simulink model "focVelocityEncoder"  (R2020a)
settings: configuration reference "EC" (kept outside this file)
model workspace (MAT data in the model file):
  PolePairs = 4
  activeLoop = 1
  statusAutotuner = 0
undefined symbols (not defined in the file): adcTransducerVoltAtZeroAmpere, adcTransducerVoltPerAmpere, DiscIntNeverNeededParam, encoderCalibrationDuration, encoderCalibrationVoltage, encoderCountPerRevolution, inverterBusVoltage, inverterCurrentMax, paramCurrentControlI, paramCurrentControlP, paramOpenLoopVelocityAcceleration, paramOpenLoopVelocityToVoltsBias, paramOpenLoopVelocityToVoltsScalar, paramOverCurrentEnable, paramVelocityControlI, paramVelocityControlP, pwmComparePerVolt, pwmCounterMax, sampleTimeCurrentControl
libraries: mcbcontrolslib x12, simulink x7, mcbpositiondecoderlib x4, focautotunershared x1
settings Model: DataDictionary=controllerData.sldd  EnableAccessToBaseWorkspace=off  ParameterArgumentNames=PolePairs,activeLoop,statusAutotuner  OrderedModelArguments=off  Creator=The MathWorks, Inc.  LastModifiedBy=manuel.fedou
settings ConfigSetRef: SourceName=EC

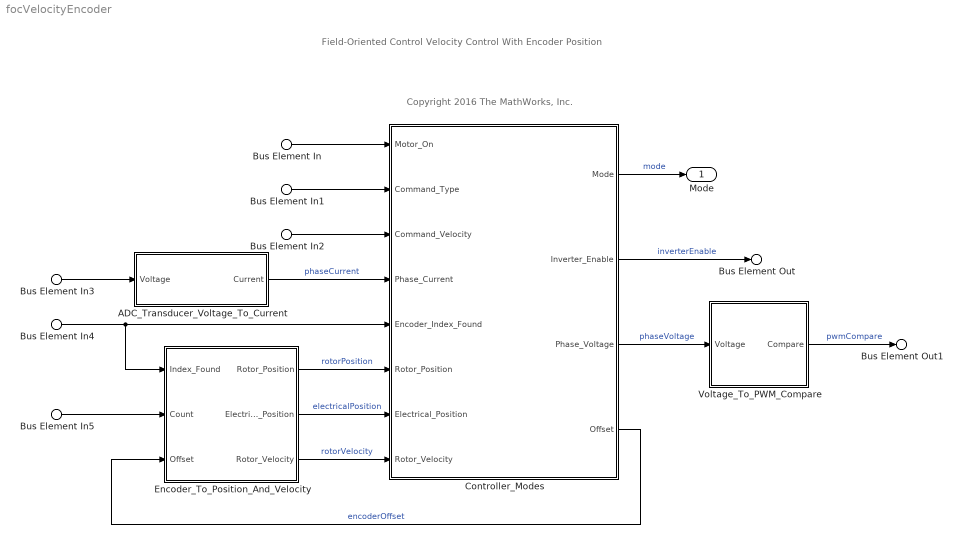
== system focVelocityEncoder ==
  note: Field-Oriented Control
      | Velocity Control With Encoder Position
  note: Copyright 2016 The MathWorks, Inc.
  Bus Element In : Inport  PortName=inputs  Element=motorOn
  Bus Element In1 : Inport  PortName=inputs  Element=commandType
  Bus Element In2 : Inport  PortName=inputs  Element=velocityCommand
  Bus Element In3 : Inport  Port=2  PortName=feedback  Element=transducerVoltage
  Bus Element In4 : Inport  Port=2  PortName=feedback  Element=encoderIndexFound
  Bus Element In5 : Inport  Port=2  PortName=feedback  Element=encoderCount
  ADC_Transducer_Voltage_To_Current : Subsystem
  Controller_Modes : Subsystem
  Encoder_To_Position_And_Velocity : Subsystem  VariantControl=isMCB == 1
  Voltage_To_PWM_Compare : Subsystem
  Mode : Outport  PortDimensions=1  VectorParamsAs1DForOutWhenUnconnected=off
  Bus Element Out : Outport  Port=2  PortName=commands  Element=inverterEnable
  Bus Element Out1 : Outport  Port=2  PortName=commands  Element=pwmCompare
  wires:
  ADC_Transducer_Voltage_To_Current/1(Current) -> Controller_Modes/4(Phase_Current)  "phaseCurrent"
  Controller_Modes/4(Offset) -> Encoder_To_Position_And_Velocity/3(Offset)  "encoderOffset"
  Bus Element In4/1 -> Encoder_To_Position_And_Velocity/1(Index_Found), Controller_Modes/5(Encoder_Index_Found)
  Voltage_To_PWM_Compare/1(Compare) -> Bus Element Out1/1  "pwmCompare"
  Bus Element In3/1 -> ADC_Transducer_Voltage_To_Current/1(Voltage)
  Controller_Modes/1(Mode) -> Mode/1  "mode"
  Controller_Modes/3(Phase_Voltage) -> Voltage_To_PWM_Compare/1(Voltage)  "phaseVoltage"
  Controller_Modes/2(Inverter_Enable) -> Bus Element Out/1  "inverterEnable"
  Bus Element In5/1 -> Encoder_To_Position_And_Velocity/2(Count)
  Encoder_To_Position_And_Velocity/1(Rotor_Position) -> Controller_Modes/6(Rotor_Position)  "rotorPosition"
  Encoder_To_Position_And_Velocity/2(Electrical_Position) -> Controller_Modes/7(Electrical_Position)  "electricalPosition"
  Encoder_To_Position_And_Velocity/3(Rotor_Velocity) -> Controller_Modes/8(Rotor_Velocity)  "rotorVelocity"
  Bus Element In1/1 -> Controller_Modes/2(Command_Type)
  Bus Element In/1 -> Controller_Modes/1(Motor_On)
  Bus Element In2/1 -> Controller_Modes/3(Command_Velocity)

== system focVelocityEncoder/ADC_Transducer_Voltage_To_Current ==
  note: ADC Transducer Voltage to Current
  Voltage : Inport
  Add : Sum  Inputs=+-
  Bias_To_Remove : Constant  Value=adcTransducerVoltAtZeroAmpere  OutDataTypeStr=Inherit: Inherit via back propagation  SampleTime=-1
  Divide : Product  Inputs=*/
  Scalar : Constant  Value=adcTransducerVoltPerAmpere  OutDataTypeStr=Inherit: Inherit via back propagation  SampleTime=-1
  Current : Outport  VectorParamsAs1DForOutWhenUnconnected=off
  wires:
  Voltage/1 -> Add/1
  Add/1 -> Divide/1
  Scalar/1 -> Divide/2
  Divide/1 -> Current/1
  Bias_To_Remove/1 -> Add/2

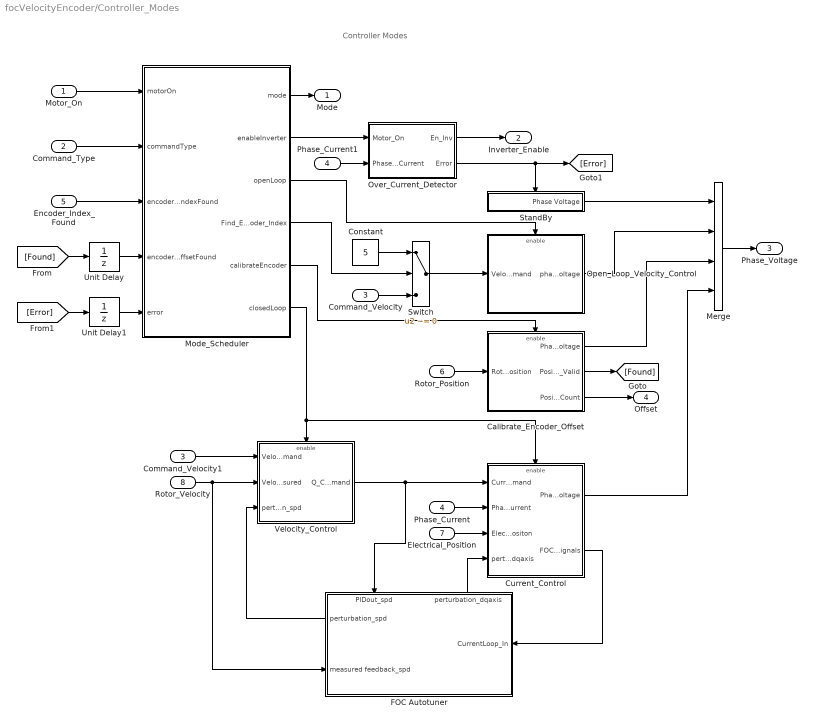
== system focVelocityEncoder/Controller_Modes ==
  note: Controller Modes
  Motor_On : Inport
  Command_Type : Inport  Port=2
  Command_Velocity : Inport  Port=3
  Phase_Current : Inport  Port=4
  Encoder_Index_Found : Inport  Port=5
  Rotor_Position : Inport  Port=6
  Electrical_Position : Inport  Port=7
  Rotor_Velocity : Inport  Port=8
  Calibrate_Encoder_Offset : Subsystem
      mask Display: fprintf('Calibrate\nEncoder\nOffset')
  Command_Velocity1 : InportShadow  Port=3
  Constant : Constant  Value=5  OutDataTypeStr=Inherit: Inherit via back propagation  SampleTime=-1
  Current_Control : Subsystem
      mask Display: fprintf('Current\nControl')
  FOC Autotuner : Subsystem  Variant=on  VariantControlMode=Label  VariantControl=Choice  LabelModeActiveChoice=dummyVariant
      settings: PortSchema="{\"entries\":[{\"content\":{\"sides\":[{\"content\":{\"connectorIds\":[\"Out2\",\"In1\"]},\"type\":\"ConnectorPlacement.EquallySpacedRectSide\",\"uuid\":\"a8b69d11-b8b6-4c45-a37c-f2894d64c9bb\"},{\"content\":{\"connectorIds\":[\"In3\"],\"side\":\"RIGHT\"},\"type\":\"ConnectorPlacement.EquallySpacedRectSide\",\"uuid\":\"22efc6fa-b445-4d82-b4a6-fe483b816bd6\"},{\"content\":{\"connectorIds\":[\"In2\",\"Out1\"],\"side\":\"TOP\"},\"type\":\"ConnectorPlacement.EquallySpacedRectSide\",\"uuid\":\"13837f3f-03ad-4a4a-a1cf-81e26a9a881f\"}]},\"type\":\"ConnectorPlacement.EquallySpacedConnector\",\"uuid\":\"91c3fe0f-f3e7-4ad7-9fa7-cccbc8809dba\"}],\"packageUris\":[\"http://schema.mathworks.com/mf0/Connector/19700101\"],\"version\":\"1.0\"}"
  Merge : Merge  Inputs=4
      mask Display: fprintf(' ')
  Mode_Scheduler : Stateflow chart  TreatAsAtomicUnit=on
  Open_Loop_Velocity_Control : Subsystem  TreatAsAtomicUnit=on
      settings: RTWFcnNameOpts=User specified  FunctionInterfaceSpec=Allow arguments (Optimized)
      mask Display: fprintf('Open Loop\nVelocity\nControl')
  Over_Current_Detector : Subsystem  TreatAsAtomicUnit=on
      mask Display: fprintf('Detect\nOvercurrent')
  Phase_Current1 : InportShadow  Port=4
  StandBy : Subsystem  Description=Stand By mode for controller outputs constant phase voltages.  TreatAsAtomicUnit=on
      mask Display: fprintf('Disabled')
  Switch : Switch  Criteria=u2 ~= 0
  Unit Delay : UnitDelay  SampleTime=-1  HasFrameUpgradeWarning=on
  Unit Delay1 : UnitDelay  SampleTime=-1  HasFrameUpgradeWarning=on
  Velocity_Control : Subsystem
      mask Display: fprintf('Velocity\nControl')
  Mode : Outport  VectorParamsAs1DForOutWhenUnconnected=off
  Inverter_Enable : Outport  Port=2  VectorParamsAs1DForOutWhenUnconnected=off
  Phase_Voltage : Outport  Port=3  VectorParamsAs1DForOutWhenUnconnected=off
  Offset : Outport  Port=4  VectorParamsAs1DForOutWhenUnconnected=off
  wires:
  Calibrate_Encoder_Offset/2(Position_At_Zero_Count_Valid) -> [Found]
  Phase_Current1/1 -> Over_Current_Detector/2(Phase_Current)
  Mode_Scheduler/2(" enableInverter") -> Over_Current_Detector/1(Motor_On)
  Merge/1 -> Phase_Voltage/1
  Calibrate_Encoder_Offset/3(Position_At_Zero_Count) -> Offset/1
  Rotor_Position/1 -> Calibrate_Encoder_Offset/1(Rotor_Position)
  Calibrate_Encoder_Offset/1(Phase_Voltage) -> Merge/3
  StandBy/1(Phase Voltage) -> Merge/1
  Mode_Scheduler/5(" calibrateEncoder") -> Calibrate_Encoder_Offset/Enable
  Switch/1 -> Open_Loop_Velocity_Control/1(Velocity_Command)
  Open_Loop_Velocity_Control/1(phase_voltage) -> Merge/2
  Current_Control/1(Phase_Voltage) -> Merge/4
  Phase_Current/1 -> Current_Control/2(Phase_Current)
  Electrical_Position/1 -> Current_Control/3(Electrical_Positon)
  Mode_Scheduler/3(" openLoop") -> Open_Loop_Velocity_Control/Enable
  Rotor_Velocity/1 -> Velocity_Control/2(Velocity_Measured), FOC Autotuner/1(measured feedback_spd)
  Over_Current_Detector/1(En_Inv) -> Inverter_Enable/1
  Command_Type/1 -> Mode_Scheduler/2(commandType)
  Motor_On/1 -> Mode_Scheduler/1(motorOn)
  [Error] -> Unit Delay1/1
  [Found] -> Unit Delay/1
  Encoder_Index_Found/1 -> Mode_Scheduler/3(encoderIndexFound)
  Mode_Scheduler/1(mode) -> Mode/1
  FOC Autotuner/1(perturbation_dqaxis) -> Current_Control/4(perturbation_dqaxis)
  Current_Control/2(FOC_Autotuner_Signals) -> FOC Autotuner/3(CurrentLoop_In)
  FOC Autotuner/2(perturbation_spd) -> Velocity_Control/3(perturbation_spd)
  Velocity_Control/1(Q_Current_Command) -> Current_Control/1(Current_Command), FOC Autotuner/2(PIDout_spd)
  Mode_Scheduler/4(" Find_Encoder_Index") -> Switch/2
  Command_Velocity/1 -> Switch/3
  Constant/1 -> Switch/1
  Over_Current_Detector/2(Error) -> StandBy/Enable, [Error]
  Command_Velocity1/1 -> Velocity_Control/1(Velocity_Command)
  Unit Delay/1 -> Mode_Scheduler/4(encoderOffsetFound)
  Unit Delay1/1 -> Mode_Scheduler/5(error)
  Mode_Scheduler/6(" closedLoop") -> Velocity_Control/Enable, Current_Control/Enable

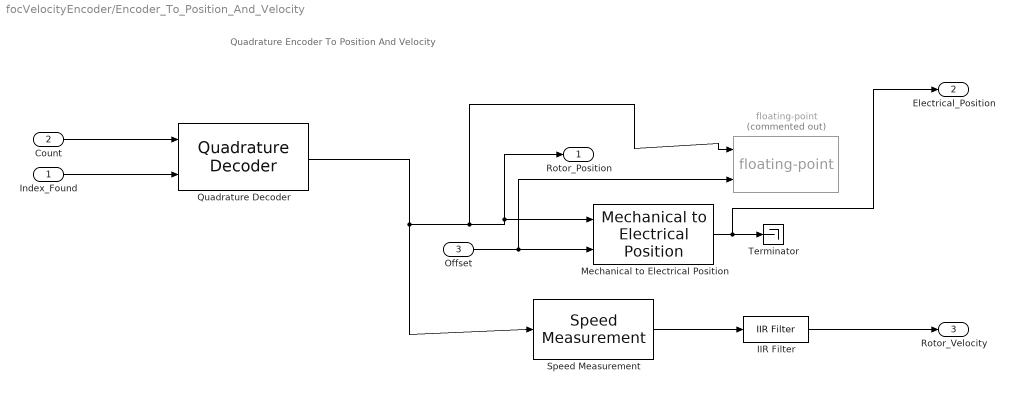
== system focVelocityEncoder/Encoder_To_Position_And_Velocity ==
  note: Quadrature Encoder To Position And Velocity
  Index_Found : Inport
  Count : Inport  Port=2
  Offset : Inport  Port=3
  IIR Filter : mcbcontrolslib/IIR Filter  Filter_constant=0.01
      settings: SourceProductBaseCode=MT
  Mechanical to Electrical Position : mcbpositiondecoderlib/Mechanical to Electrical Position  LabelModeActiveChoice=floating-point  NrPP=7  selectedRange=Radians  MechOfstInputType=Input port  mechOffsetIn=0  maxAngleIn=2*pi  InputDataType=single  VariantSelect=floating-point
      settings: SourceProductBaseCode=MT
  Quadrature Decoder : mcbpositiondecoderlib/Quadrature Decoder  EncoderSlitsPerRevolution=1024  EncoderCountsPerSlit=4  CounterSize=16 bits  ExternalIndexCount=on  PositionUnit=Radians  PositionDataType=single
      settings: SourceProductBaseCode=MT
  Speed Measurement : mcbpositiondecoderlib/Speed Measurement  PositionUnit=Radians  SpeedCalculationMode=Maximum application speed  SampleTimeAsync=0.0002  MaximumApplicationSpeed=5000  SpeedResolution=3  DelayLength=29  MaximumMeasurableSpeed=5000  MeasurableSpeedResolution=2.3283e-06  SpeedUnit=Radians/Sec  PerUnitSpeed=1000  SpeedDataType=single
      settings: SourceProductBaseCode=MT
  Terminator : Terminator
  floating-point : mcbpositiondecoderlib/Mechanical to Electrical Position/floating-point  Commented=on  SystemSampleTime=-1  VariantControl=floating-point  Latency=0  AutoFrameSizeCalculation=off
      settings: SourceProductBaseCode=MT
  Rotor_Position : Outport  VectorParamsAs1DForOutWhenUnconnected=off
  Electrical_Position : Outport  Port=2  VectorParamsAs1DForOutWhenUnconnected=off
  Rotor_Velocity : Outport  Port=3  VectorParamsAs1DForOutWhenUnconnected=off
  wires:
  Index_Found/1 -> Quadrature Decoder/2
  Count/1 -> Quadrature Decoder/1
  Speed Measurement/1 -> IIR Filter/1
  IIR Filter/1 -> Rotor_Velocity/1
  Offset/1 -> floating-point/2, Mechanical to Electrical Position/2
  Quadrature Decoder/1 -> Mechanical to Electrical Position/1, Rotor_Position/1, floating-point/1, Speed Measurement/1
  Mechanical to Electrical Position/1 -> Electrical_Position/1, Terminator/1

== system focVelocityEncoder/Voltage_To_PWM_Compare ==
  note: Voltage To PWM Compare
  Voltage : Inport
  Bias1 : Bias  Bias=pwmCounterMax/2
  Data_Type_Conversion : DataTypeConversion  OutDataTypeStr=uint16  LockScale=on
  Saturation : Saturate  UpperLimit=pwmCounterMax  LowerLimit=0
      settings: AttributesFormatString=|
      | --------------------------------
      | Upper Limit = %<UpperLimit>
      | Lower Limit = %<LowerLimit>
  Slope : Gain  Gain=pwmComparePerVolt
      settings: AttributesFormatString=|
      | ----------------------------------------
      | Gain = %<Gain>
  Compare : Outport  VectorParamsAs1DForOutWhenUnconnected=off
  wires:
  Saturation/1 -> Data_Type_Conversion/1
  Voltage/1 -> Slope/1  "phaseVoltage"
  Data_Type_Conversion/1 -> Compare/1  "pwmCompare"
  Slope/1 -> Bias1/1
  Bias1/1 -> Saturation/1

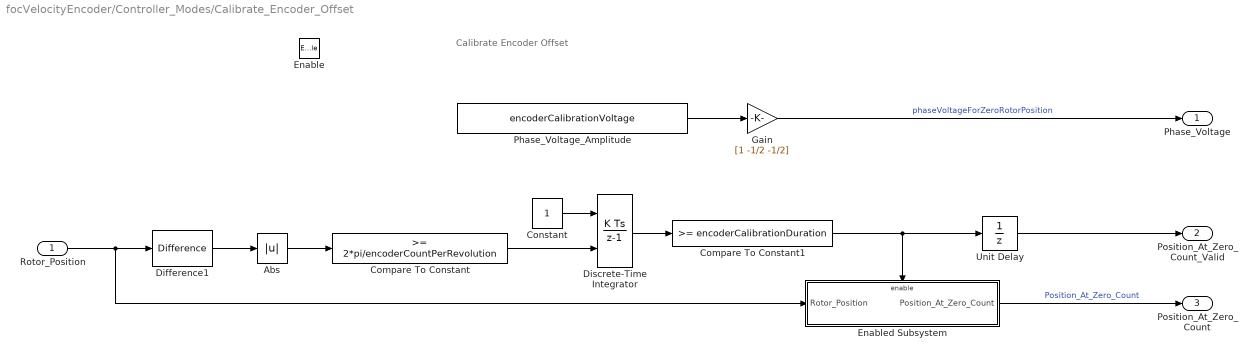
== system focVelocityEncoder/Controller_Modes/Calibrate_Encoder_Offset ==
  note: Calibrate Encoder Offset
  Rotor_Position : Inport  PortDimensions=1  Interpolate=off
  Enable : EnablePort  StatesWhenEnabling=reset
      settings: AttributesFormatString=|
      | ----------------------------------------
      | States when enabling = %<StatesWhenEnabling>
  Abs : Abs
  Compare To Constant : simulink/Logic and Bit Operations/Compare To Constant  relop=>=  const=2*pi/encoderCountPerRevolution  OutDataTypeStr=boolean
  Compare To Constant1 : simulink/Logic and Bit Operations/Compare To Constant  relop=>=  const=encoderCalibrationDuration  OutDataTypeStr=boolean
  Constant : Constant
  Difference1 : simulink/Discrete/Difference  ICPrevInput=0.0  OutMin=[]  OutMax=[]  OutDataType=fixdt(1, 16)  OutScaling=2^-10  DoSatur=off
  Discrete-Time Integrator : DiscreteIntegrator  ExternalReset=rising  SampleTime=-1  ICPrevOutput=DiscIntNeverNeededParam  ICPrevScaledInput=DiscIntNeverNeededParam
  Enabled Subsystem : Subsystem  TreatAsAtomicUnit=on
  Gain : Gain  Gain=[1 -1/2 -1/2]
      settings: AttributesFormatString=|
      | ----------------------------------
      | Gain = %<Gain>
  Phase_Voltage_Amplitude : Constant  Value=encoderCalibrationVoltage  OutDataTypeStr=Inherit: Inherit via back propagation
  Unit Delay : UnitDelay  SampleTime=-1  HasFrameUpgradeWarning=on
  Phase_Voltage : Outport  PortDimensions=3  SourceOfInitialOutputValue=Input signal  InitialOutput=0  VectorParamsAs1DForOutWhenUnconnected=off
  Position_At_Zero_Count_Valid : Outport  Port=2  OutputWhenDisabled=reset  InitialOutput=0  VectorParamsAs1DForOutWhenUnconnected=off
  Position_At_Zero_Count : Outport  Port=3  SourceOfInitialOutputValue=Input signal  VectorParamsAs1DForOutWhenUnconnected=off
  wires:
  Unit Delay/1 -> Position_At_Zero_Count_Valid/1
  Enabled Subsystem/1(Position_At_Zero_Count) -> Position_At_Zero_Count/1  "Position_At_Zero_Count"
  Discrete-Time Integrator/1 -> Compare To Constant1/1
  Constant/1 -> Discrete-Time Integrator/1
  Abs/1 -> Compare To Constant/1
  Difference1/1 -> Abs/1
  Compare To Constant/1 -> Discrete-Time Integrator/2
  Gain/1 -> Phase_Voltage/1  "phaseVoltageForZeroRotorPosition"
  Phase_Voltage_Amplitude/1 -> Gain/1
  Rotor_Position/1 -> Enabled Subsystem/1(Rotor_Position), Difference1/1
  Compare To Constant1/1 -> Unit Delay/1, Enabled Subsystem/Enable

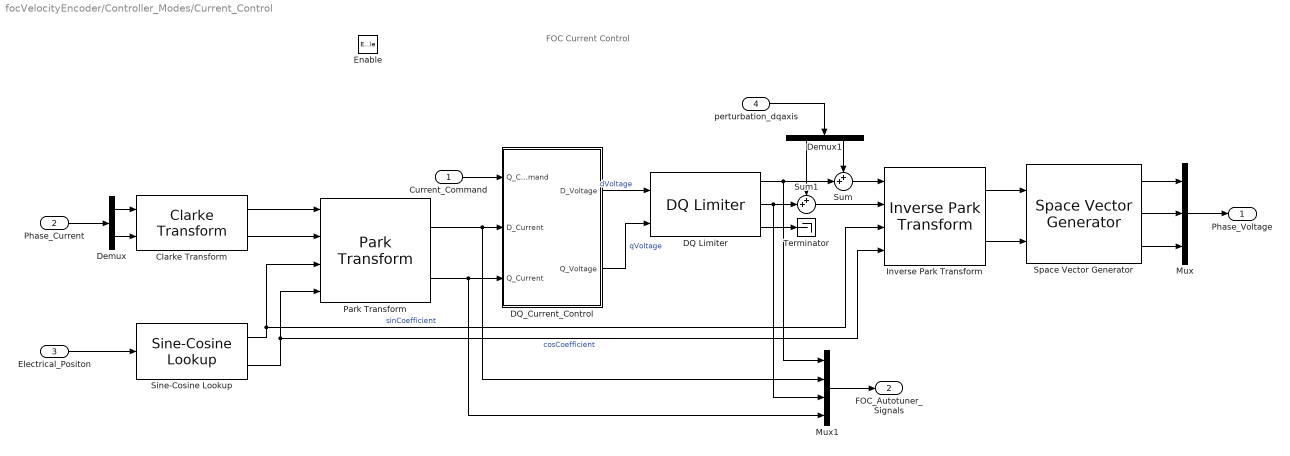
== system focVelocityEncoder/Controller_Modes/Current_Control ==
  note: FOC Current Control
  Current_Command : Inport
  Phase_Current : Inport  Port=2
  Electrical_Positon : Inport  Port=3
  perturbation_dqaxis : Inport  Port=4
  Enable : EnablePort  StatesWhenEnabling=reset
      settings: AttributesFormatString=|
      | ----------------------------------------
      | States when enabling = %<StatesWhenEnabling>
  Clarke Transform : mcbcontrolslib/Clarke Transform  VariantControl=Variant2
  DQ Limiter : mcbcontrolslib/DQ Limiter  Vmax=inverterBusVoltage/sqrt(3)
      settings: SourceProductBaseCode=MT
  DQ_Current_Control : Subsystem
  Demux : Demux  Outputs=2
  Demux1 : Demux  Outputs=2
  Inverse Park Transform : mcbcontrolslib/Inverse Park Transform  AxisAlignment=D-axis
  Mux : Mux  Inputs=3
  Mux1 : Mux
  Park Transform : mcbcontrolslib/Park Transform  AxisAlignment=D-axis
      settings: SourceProductBaseCode=MT
  Sine-Cosine Lookup : mcbcontrolslib/Sine-Cosine Lookup  AngleInput=Radians  N_points=1024
      settings: SourceProductBaseCode=MT
  Space Vector Generator : mcbcontrolslib/Space Vector Generator
      settings: SourceProductBaseCode=MT
  Sum : Sum  Inputs=++|
  Sum1 : Sum  Inputs=++|
  Terminator : Terminator
  Phase_Voltage : Outport  SourceOfInitialOutputValue=Input signal  VectorParamsAs1DForOutWhenUnconnected=off
  FOC_Autotuner_Signals : Outport  Port=2  VectorParamsAs1DForOutWhenUnconnected=off
  wires:
  Park Transform/2 -> Mux1/4, DQ_Current_Control/3(Q_Current)
  Park Transform/1 -> Mux1/2, DQ_Current_Control/2(D_Current)
  Inverse Park Transform/2 -> Space Vector Generator/2
  Inverse Park Transform/1 -> Space Vector Generator/1
  Clarke Transform/2 -> Park Transform/2
  Clarke Transform/1 -> Park Transform/1
  Mux/1 -> Phase_Voltage/1
  Electrical_Positon/1 -> Sine-Cosine Lookup/1
  Sine-Cosine Lookup/2 -> Inverse Park Transform/4, Park Transform/4  "cosCoefficient"
  Sine-Cosine Lookup/1 -> Inverse Park Transform/3, Park Transform/3  "sinCoefficient"
  Demux/1 -> Clarke Transform/1
  Demux/2 -> Clarke Transform/2
  Phase_Current/1 -> Demux/1
  Space Vector Generator/1 -> Mux/1
  Space Vector Generator/2 -> Mux/2
  Space Vector Generator/3 -> Mux/3
  DQ_Current_Control/1(D_Voltage) -> DQ Limiter/1  "dVoltage"
  DQ_Current_Control/2(Q_Voltage) -> DQ Limiter/2  "qVoltage"
  DQ Limiter/3 -> Terminator/1
  Sum/1 -> Inverse Park Transform/1
  DQ Limiter/1 -> Mux1/1, Sum/2
  DQ Limiter/2 -> Mux1/3, Sum1/2
  Sum1/1 -> Inverse Park Transform/2
  Demux1/1 -> Sum1/1
  Demux1/2 -> Sum/1
  perturbation_dqaxis/1 -> Demux1/1
  Mux1/1 -> FOC_Autotuner_Signals/1
  Current_Command/1 -> DQ_Current_Control/1(Q_Command)

== system focVelocityEncoder/Controller_Modes/FOC Autotuner ==
  measured feedback_spd : Inport
  PIDout_spd : Inport  Port=2
  CurrentLoop_In : Inport  Port=3
  Autotuner : Subsystem  VariantControl=autotunerVariant
  Dummy : Subsystem  VariantControl=dummyVariant
  perturbation_dqaxis : Outport
  perturbation_spd : Outport  Port=2

== system focVelocityEncoder/Controller_Modes/Open_Loop_Velocity_Control ==
  note: Open Loop Velocity Control
  Velocity_Command : Inport
  Enable : EnablePort  StatesWhenEnabling=reset
      settings: AttributesFormatString=|
      | ----------------------------------------
      | States when enabling = %<StatesWhenEnabling>
  3-Phase Sine Voltage Generator : mcbcontrolslib/3-Phase Sine Voltage Generator  AngleInput=Radians  N_points=1024
      settings: SourceProductBaseCode=MT
  Mux : Mux  Inputs=3
  Ramp_Velocity : Subsystem
  Rotor_Velocity_To_Volts : Subsystem
  Wrapped State DTI : Subsystem
  phase_voltage : Outport  SourceOfInitialOutputValue=Input signal  VectorParamsAs1DForOutWhenUnconnected=off
  wires:
  3-Phase Sine Voltage Generator/1 -> Mux/1
  3-Phase Sine Voltage Generator/2 -> Mux/2
  3-Phase Sine Voltage Generator/3 -> Mux/3
  Rotor_Velocity_To_Volts/1(V) -> 3-Phase Sine Voltage Generator/1  "quadratureVoltage"
  Velocity_Command/1 -> Ramp_Velocity/1(Velocity_Command)
  Ramp_Velocity/1(Rotor_Velocity) -> Rotor_Velocity_To_Volts/1(RV)
  Mux/1 -> phase_voltage/1
  Ramp_Velocity/2(Electrical_Velocity) -> Wrapped State DTI/1(Angular Speed)
  Wrapped State DTI/1(Angular Position) -> 3-Phase Sine Voltage Generator/2

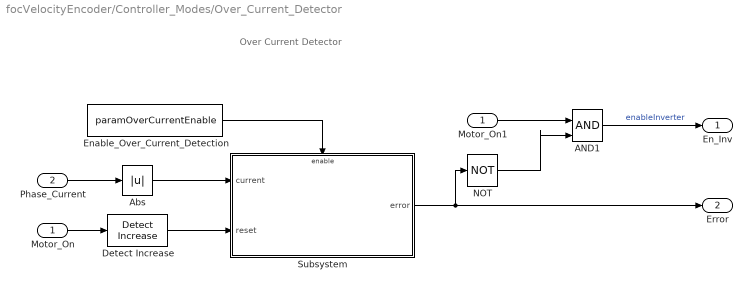
== system focVelocityEncoder/Controller_Modes/Over_Current_Detector ==
  note: Over Current Detector
  Motor_On : Inport
  Phase_Current : Inport  Port=2
  AND1 : Logic  IconShape=distinctive  AllPortsSameDT=off  OutDataTypeStr=boolean
  Abs : Abs
  Detect Increase : simulink/Logic and Bit Operations/Detect Increase  vinit=0.0  OutDataTypeStr=boolean
  Enable_Over_Current_Detection : Constant  Value=paramOverCurrentEnable
  Motor_On1 : InportShadow
  NOT : Logic  Operator=NOT  IconShape=distinctive  AllPortsSameDT=off  OutDataTypeStr=boolean
  Subsystem : Subsystem
  En_Inv : Outport  VectorParamsAs1DForOutWhenUnconnected=off
  Error : Outport  Port=2  VectorParamsAs1DForOutWhenUnconnected=off
  wires:
  Motor_On1/1 -> AND1/1
  NOT/1 -> AND1/2
  AND1/1 -> En_Inv/1  "enableInverter"
  Motor_On/1 -> Detect Increase/1
  Phase_Current/1 -> Abs/1
  Subsystem/1(error) -> Error/1, NOT/1
  Abs/1 -> Subsystem/1(current)
  Detect Increase/1 -> Subsystem/2(reset)
  Enable_Over_Current_Detection/1 -> Subsystem/Enable

== system focVelocityEncoder/Controller_Modes/StandBy ==
  note: Disabled
  Enable : EnablePort  StatesWhenEnabling=reset
      settings: AttributesFormatString=|
      | ----------------------------------------
      | States when enabling = %<StatesWhenEnabling>
  Constant : Constant  Value=[0 0 0]  OutDataTypeStr=Inherit: Inherit via back propagation
  Phase Voltage : Outport  SourceOfInitialOutputValue=Input signal  VectorParamsAs1DForOutWhenUnconnected=off
  wires:
  Constant/1 -> Phase Voltage/1

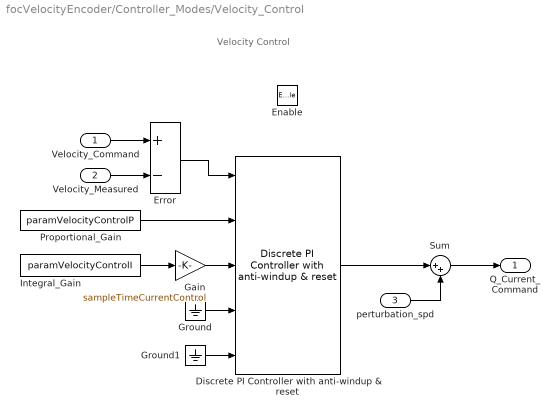
== system focVelocityEncoder/Controller_Modes/Velocity_Control ==
  note: Velocity Control
  Velocity_Command : Inport
  Velocity_Measured : Inport  Port=2
  perturbation_spd : Inport  Port=3
  Enable : EnablePort  StatesWhenEnabling=reset
      settings: AttributesFormatString=|
      | ----------------------------------------
      | States when enabling = %<StatesWhenEnabling>
  Discrete PI Controller with anti-windup & reset : mcbcontrolslib/Discrete PI Controller  with anti-windup & reset  UpperSaturationLimit=inverterCurrentMax  LowerSaturationLimit=-inverterCurrentMax
      settings: SourceProductBaseCode=MT
  Error : Sum  Inputs=+-
  Gain : Gain  Gain=sampleTimeCurrentControl
  Ground : Ground
  Ground1 : Ground
  Integral_Gain : Constant  Value=paramVelocityControlI  OutDataTypeStr=Inherit: Inherit via back propagation
  Proportional_Gain : Constant  Value=paramVelocityControlP  OutDataTypeStr=Inherit: Inherit via back propagation
  Sum : Sum  Inputs=|++
  Q_Current_Command : Outport  SourceOfInitialOutputValue=Input signal  InitialOutput=0  VectorParamsAs1DForOutWhenUnconnected=off
  wires:
  Proportional_Gain/1 -> Discrete PI Controller with anti-windup & reset/2
  Velocity_Command/1 -> Error/1
  Velocity_Measured/1 -> Error/2
  Error/1 -> Discrete PI Controller with anti-windup & reset/1
  Gain/1 -> Discrete PI Controller with anti-windup & reset/3
  Integral_Gain/1 -> Gain/1
  Discrete PI Controller with anti-windup & reset/1 -> Sum/1
  Sum/1 -> Q_Current_Command/1
  perturbation_spd/1 -> Sum/2
  Ground/1 -> Discrete PI Controller with anti-windup & reset/4
  Ground1/1 -> Discrete PI Controller with anti-windup & reset/5

== system focVelocityEncoder/Controller_Modes/Calibrate_Encoder_Offset/Enabled Subsystem ==
  Rotor_Position : Inport
  Enable : EnablePort
  Position_At_Zero_Count : Outport  SourceOfInitialOutputValue=Input signal  InitialOutput=0
  wires:
  Rotor_Position/1 -> Position_At_Zero_Count/1

== system focVelocityEncoder/Controller_Modes/Current_Control/DQ_Current_Control ==
  note: DQ Current Control
  Q_Command : Inport
  D_Current : Inport  Port=2
  Q_Current : Inport  Port=3
  D_Command : Constant  Value=0  OutDataTypeStr=Inherit: Inherit via back propagation
  D_Current_Control : Subsystem
  Q_Current_Control : Subsystem
  D_Voltage : Outport  VectorParamsAs1DForOutWhenUnconnected=off
  Q_Voltage : Outport  Port=2  VectorParamsAs1DForOutWhenUnconnected=off
  wires:
  D_Current/1 -> D_Current_Control/2(Current_Measured)
  Q_Current/1 -> Q_Current_Control/2(Current_Measured)
  D_Current_Control/1(Voltage) -> D_Voltage/1
  Q_Current_Control/1(Voltage) -> Q_Voltage/1
  Q_Command/1 -> Q_Current_Control/1(Current_Command)
  D_Command/1 -> D_Current_Control/1(Current_Command)

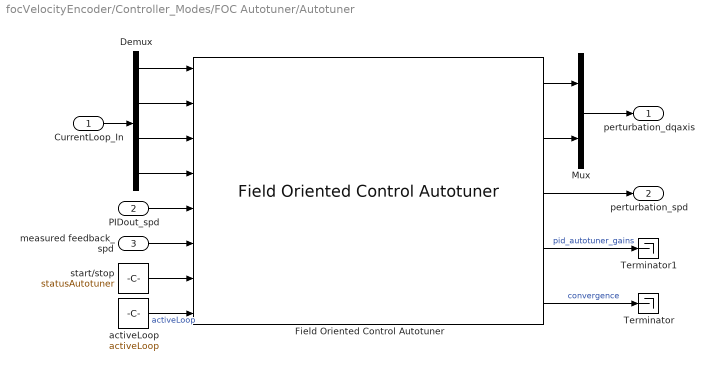
== system focVelocityEncoder/Controller_Modes/FOC Autotuner/Autotuner ==
  CurrentLoop_In : Inport
  PIDout_spd : Inport  Port=2
  measured feedback_spd : Inport  Port=3
  Demux : Demux
  Field Oriented Control Autotuner : focautotunershared/Field Oriented Control Autotuner  TuneDaxisLoop=on  TuneQaxisLoop=on  TuneSpeedLoop=on  TuneFluxLoop=off  UseSameSettingsInner=off  UseSameSettingsOuter=off  TimeDomain=discrete-time  PIDTypeAllInner=PI  PIDFormAllInner=Parallel  TsAllInner=0.001  IntegratorMethodAllInner=Forward Euler  FilterMethodAllInner=Forward Euler  BandwidthAllInner=100  TargetPMAllInner=60  PIDTypeDaxis=PI  PIDFormDaxis=Parallel  TsDaxis=-1  IntegratorMethodDaxis=Forward Euler  FilterMethodDaxis=Forward Euler  BandwidthDaxis=100  TargetPMDaxis=60  PIDTypeQaxis=PI  PIDFormQaxis=Parallel  TsQaxis=-1  IntegratorMethodQaxis=Forward Euler  FilterMethodQaxis=Forward Euler  BandwidthQaxis=100  TargetPMQaxis=60  PIDTypeAllOuter=PI  PIDFormAllOuter=Parallel  TsAllOuter=0.1  IntegratorMethodAllOuter=Forward Euler  FilterMethodAllOuter=Forward Euler  BandwidthAllOuter=1  TargetPMAllOuter=60  PIDTypeSpeed=PI  PIDFormSpeed=Parallel  TsSpeed=-1  IntegratorMethodSpeed=Forward Euler  FilterMethodSpeed=Forward Euler  BandwidthSpeed=2  TargetPMSpeed=60  PIDTypeFlux=PI  PIDFormFlux=Parallel  TsFlux=0.1  IntegratorMethodFlux=Forward Euler  FilterMethodFlux=Forward Euler  BandwidthFlux=1  TargetPMFlux=60  StartTimeDaxis=1  DurationDaxis=0.05  StopTimeDaxis=1.05  StartTimeQaxis=1.1  DurationQaxis=0.05  StopTimeQaxis=1.15  StartTimeSpeed=2  DurationSpeed=3  StopTimeSpeed=5  StartTimeFlux=6  DurationFlux=3  StopTimeFlux=9  PlantTypeAllInner=Stable  PlantSignAllInner=Positive  AmpSineAllInner=1  PlantTypeDaxis=Stable  PlantSignDaxis=Positive  AmpSineDaxis=1  PlantTypeQaxis=Stable  PlantSignQaxis=Positive  AmpSineQaxis=1  PlantTypeAllOuter=Stable  PlantSignAllOuter=Positive  AmpSineAllOuter=1  PlantTypeSpeed=Stable  PlantSignSpeed=Positive  AmpSineSpeed=10  PlantTypeFlux=Stable  PlantSignFlux=Positive  AmpSineFlux=1  UseExternalWc=off  UseExternalPM=off  UseExternalSourceStartStop=on  UseExternalAmpSine=off  UseExternalAchievedPM=off  UseExternalFRD=off  UseExternalU0=off  UseExternalActiveLoop=off  BlockDataType=single  variantStartStop=variantExternal  variantBandwidth=variantInternal  variantPhaseMargin=variantInternal  variantSineAmplitudes=variantInternal  variantEnableDaxis=variantLoopEnabled  variantEnableQaxis=variantLoopEnabled  variantEnableSpeed=variantLoopEnabled  variantEnableFlux=variantLoopDisabled  variantBandwidthDaxis=variantExternal  variantBandwidthQaxis=variantExternal  variantBandwidthSpeed=variantExternal  variantBandwidthFlux=variantExternal  focMode=focMode  EstimationWindowSize=3
      settings: SourceProductBaseCode=CT,ID,MT,SO
  Mux : Mux  Inputs=2
  Terminator : Terminator
  Terminator1 : Terminator
  activeLoop : Constant  Value=activeLoop
  start/stop : Constant  Value=statusAutotuner
  perturbation_dqaxis : Outport
  perturbation_spd : Outport  Port=2
  wires:
  Field Oriented Control Autotuner/4 -> Terminator1/1  "pid_autotuner_gains"
  Field Oriented Control Autotuner/1 -> Mux/1
  Field Oriented Control Autotuner/5 -> Terminator/1  "convergence"
  Demux/1 -> Field Oriented Control Autotuner/1
  Demux/4 -> Field Oriented Control Autotuner/4
  PIDout_spd/1 -> Field Oriented Control Autotuner/5
  Mux/1 -> perturbation_dqaxis/1
  measured feedback_spd/1 -> Field Oriented Control Autotuner/6
  Field Oriented Control Autotuner/2 -> Mux/2
  Demux/2 -> Field Oriented Control Autotuner/2
  Demux/3 -> Field Oriented Control Autotuner/3
  start/stop/1 -> Field Oriented Control Autotuner/7
  Field Oriented Control Autotuner/3 -> perturbation_spd/1
  activeLoop/1 -> Field Oriented Control Autotuner/8  "activeLoop"
  CurrentLoop_In/1 -> Demux/1

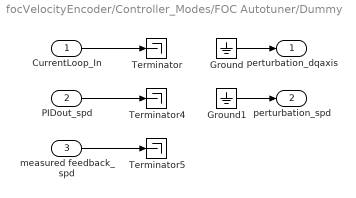
== system focVelocityEncoder/Controller_Modes/FOC Autotuner/Dummy ==
  CurrentLoop_In : Inport
  PIDout_spd : Inport  Port=2
  measured feedback_spd : Inport  Port=3
  Ground : Ground
  Ground1 : Ground
  Terminator : Terminator
  Terminator4 : Terminator
  Terminator5 : Terminator
  perturbation_dqaxis : Outport
  perturbation_spd : Outport  Port=2
  wires:
  CurrentLoop_In/1 -> Terminator/1
  PIDout_spd/1 -> Terminator4/1
  measured feedback_spd/1 -> Terminator5/1
  Ground/1 -> perturbation_dqaxis/1
  Ground1/1 -> perturbation_spd/1

== system focVelocityEncoder/Controller_Modes/Open_Loop_Velocity_Control/Ramp_Velocity ==
  note: Ramp Velocity
  Velocity_Command : Inport
  Gain : Gain  Gain=sampleTimeCurrentControl  OutDataTypeStr=Inherit: Same as input
      settings: AttributesFormatString=------------------------------\nGain = %<Gain>
  Number_Of_Pole_Pairs : Gain  Gain=PolePairs
      settings: AttributesFormatString=------------------------------------\nGain = %<Gain>
  Set_Acceleration : Subsystem
  Sum : Sum  Inputs=|++
  Unit Delay : UnitDelay  SampleTime=-1  HasFrameUpgradeWarning=on
  Rotor_Velocity : Outport  VectorParamsAs1DForOutWhenUnconnected=off
  Electrical_Velocity : Outport  Port=2  VectorParamsAs1DForOutWhenUnconnected=off
  wires:
  Velocity_Command/1 -> Set_Acceleration/1(V_Target)
  Set_Acceleration/1(accelCommand) -> Gain/1  "accelCommand"
  Number_Of_Pole_Pairs/1 -> Electrical_Velocity/1
  Gain/1 -> Sum/1  "deltaVelocityCommand"
  Unit Delay/1 -> Sum/2, Set_Acceleration/2(V_Current)
  Sum/1 -> Rotor_Velocity/1, Number_Of_Pole_Pairs/1, Unit Delay/1  "velocityCommand"

== system focVelocityEncoder/Controller_Modes/Open_Loop_Velocity_Control/Rotor_Velocity_To_Volts ==
  note: Rotor Velocity To Volts
  RV : Inport
  Abs : Abs
  Bias : Bias  Bias=paramOpenLoopVelocityToVoltsBias
  Frequency_To_Voltage : Gain  Gain=paramOpenLoopVelocityToVoltsScalar
      settings: AttributesFormatString=--------------------------------\n%<Gain>
  V : Outport  VectorParamsAs1DForOutWhenUnconnected=off
  wires:
  RV/1 -> Abs/1
  Frequency_To_Voltage/1 -> Bias/1
  Bias/1 -> V/1
  Abs/1 -> Frequency_To_Voltage/1

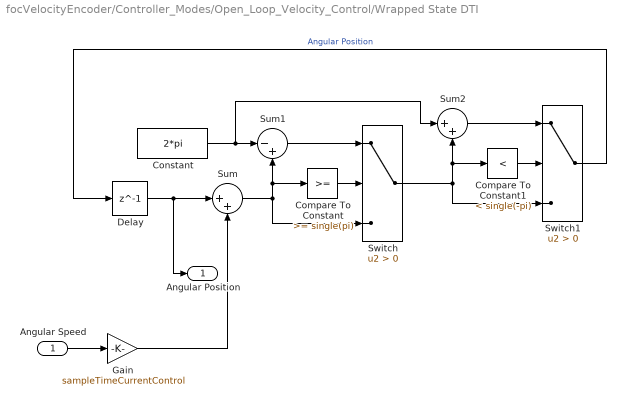
== system focVelocityEncoder/Controller_Modes/Open_Loop_Velocity_Control/Wrapped State DTI ==
  Angular Speed : Inport
  Compare To Constant : simulink/Logic and Bit Operations/Compare To Constant  relop=>=  const=single(pi)  OutDataTypeStr=boolean
  Compare To Constant1 : simulink/Logic and Bit Operations/Compare To Constant  relop=<  const=single(-pi)  OutDataTypeStr=boolean
  Constant : Constant  Value=2*pi  OutDataTypeStr=Inherit: Inherit via back propagation  SampleTime=-1
  Delay : Delay  DelayLength=1
  Gain : Gain  Gain=sampleTimeCurrentControl
  Sum : Sum  Inputs=|++
  Sum1 : Sum  Inputs=|-+
  Sum2 : Sum  Inputs=|++
  Switch : Switch  Criteria=u2 > Threshold
  Switch1 : Switch  Criteria=u2 > Threshold
  Angular Position : Outport
  wires:
  Compare To Constant1/1 -> Switch1/2
  Delay/1 -> Sum/1, Angular Position/1
  Constant/1 -> Sum2/1, Sum1/1
  Sum2/1 -> Switch1/1
  Switch1/1 -> Delay/1  "Angular Position"
  Switch/1 -> Sum2/2, Compare To Constant1/1, Switch1/3
  Compare To Constant/1 -> Switch/2
  Angular Speed/1 -> Gain/1
  Sum/1 -> Compare To Constant/1, Sum1/2, Switch/3
  Sum1/1 -> Switch/1
  Gain/1 -> Sum/2

== system focVelocityEncoder/Controller_Modes/Over_Current_Detector/Subsystem ==
  current : Inport
  reset : Inport  Port=2
  Enable : EnablePort  StatesWhenEnabling=reset
  For Iterator Subsystem : Subsystem  TreatAsAtomicUnit=on
  OR : Logic  Operator=OR  Inputs=1  AllPortsSameDT=off  OutDataTypeStr=boolean
  error : Outport  SourceOfInitialOutputValue=Input signal
  wires:
  For Iterator Subsystem/1(error) -> OR/1
  current/1 -> For Iterator Subsystem/1(current)
  OR/1 -> error/1
  reset/1 -> For Iterator Subsystem/2(reset)

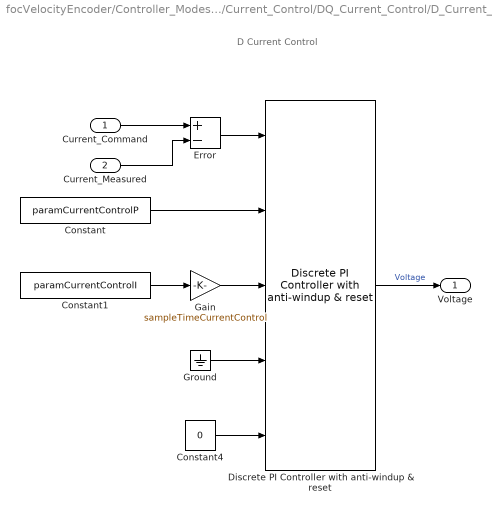
== system focVelocityEncoder/Controller_Modes/Current_Control/DQ_Current_Control/D_Current_Control ==
  note: D Current Control
  Current_Command : Inport
  Current_Measured : Inport  Port=2
  Constant : Constant  Value=paramCurrentControlP  OutDataTypeStr=Inherit: Inherit via back propagation
  Constant1 : Constant  Value=paramCurrentControlI  OutDataTypeStr=Inherit: Inherit via back propagation
  Constant4 : Constant  Value=0  OutDataTypeStr=Inherit: Inherit via back propagation
  Discrete PI Controller with anti-windup & reset : mcbcontrolslib/Discrete PI Controller  with anti-windup & reset  UpperSaturationLimit=inverterBusVoltage/sqrt(3)  LowerSaturationLimit=-inverterBusVoltage/sqrt(3)
      settings: SourceProductBaseCode=MT
  Error : Sum  Inputs=+-
  Gain : Gain  Gain=sampleTimeCurrentControl
  Ground : Ground
  Voltage : Outport  VectorParamsAs1DForOutWhenUnconnected=off
  wires:
  Current_Measured/1 -> Error/2
  Current_Command/1 -> Error/1
  Error/1 -> Discrete PI Controller with anti-windup & reset/1
  Constant/1 -> Discrete PI Controller with anti-windup & reset/2
  Discrete PI Controller with anti-windup & reset/1 -> Voltage/1  "Voltage"
  Constant4/1 -> Discrete PI Controller with anti-windup & reset/5
  Ground/1 -> Discrete PI Controller with anti-windup & reset/4
  Gain/1 -> Discrete PI Controller with anti-windup & reset/3
  Constant1/1 -> Gain/1

== system focVelocityEncoder/Controller_Modes/Current_Control/DQ_Current_Control/Q_Current_Control ==
  note: Q Current Control
  Current_Command : Inport
  Current_Measured : Inport  Port=2
  Constant : Constant  Value=paramCurrentControlP  OutDataTypeStr=Inherit: Inherit via back propagation
  Constant1 : Constant  Value=paramCurrentControlI  OutDataTypeStr=Inherit: Inherit via back propagation
  Constant4 : Constant  Value=0  OutDataTypeStr=Inherit: Inherit via back propagation
  Discrete PI Controller with anti-windup & reset : mcbcontrolslib/Discrete PI Controller  with anti-windup & reset  UpperSaturationLimit=inverterBusVoltage/sqrt(3)  LowerSaturationLimit=-inverterBusVoltage/sqrt(3)
      settings: SourceProductBaseCode=MT
  Error : Sum  Inputs=+-
  Gain : Gain  Gain=sampleTimeCurrentControl
  Ground : Ground
  Voltage : Outport  VectorParamsAs1DForOutWhenUnconnected=off
  wires:
  Discrete PI Controller with anti-windup & reset/1 -> Voltage/1  "Voltage"
  Current_Command/1 -> Error/1
  Constant/1 -> Discrete PI Controller with anti-windup & reset/2
  Gain/1 -> Discrete PI Controller with anti-windup & reset/3
  Current_Measured/1 -> Error/2
  Error/1 -> Discrete PI Controller with anti-windup & reset/1
  Ground/1 -> Discrete PI Controller with anti-windup & reset/4
  Constant4/1 -> Discrete PI Controller with anti-windup & reset/5
  Constant1/1 -> Gain/1

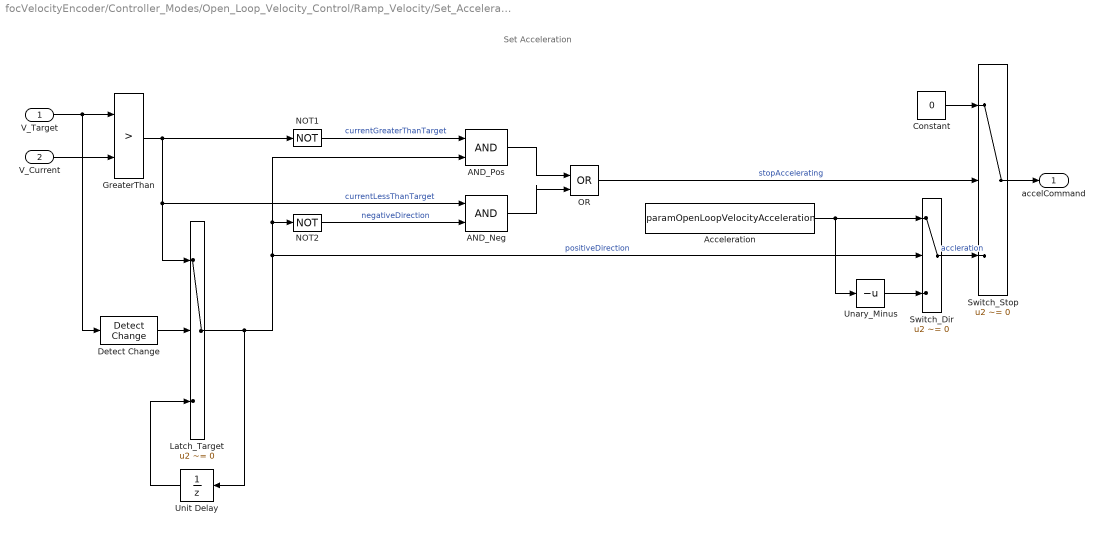
== system focVelocityEncoder/Controller_Modes/Open_Loop_Velocity_Control/Ramp_Velocity/Set_Acceleration ==
  note: Set Acceleration
  V_Target : Inport
  V_Current : Inport  Port=2
  AND_Neg : Logic  IconShape=distinctive  AllPortsSameDT=off  OutDataTypeStr=boolean
  AND_Pos : Logic  IconShape=distinctive  AllPortsSameDT=off  OutDataTypeStr=boolean
  Acceleration : Constant  Value=paramOpenLoopVelocityAcceleration  OutDataTypeStr=Inherit: Inherit via back propagation  SampleTime=-1
  Constant : Constant  Value=0  OutDataTypeStr=single
  Detect Change : simulink/Logic and Bit Operations/Detect Change  vinit=0  OutDataTypeStr=boolean
  GreaterThan : RelationalOperator  Operator=>  OutDataTypeStr=boolean  RndMeth=Simplest
  Latch_Target : Switch  Criteria=u2 ~= 0
  NOT1 : Logic  Operator=NOT  IconShape=distinctive  AllPortsSameDT=off  OutDataTypeStr=boolean
  NOT2 : Logic  Operator=NOT  IconShape=distinctive  AllPortsSameDT=off  OutDataTypeStr=boolean
  OR : Logic  Operator=OR  IconShape=distinctive  AllPortsSameDT=off  OutDataTypeStr=boolean
  Switch_Dir : Switch  Criteria=u2 ~= 0
  Switch_Stop : Switch  Criteria=u2 ~= 0
  Unary_Minus : UnaryMinus
  Unit Delay : UnitDelay  SampleTime=-1  HasFrameUpgradeWarning=on
  accelCommand : Outport  VectorParamsAs1DForOutWhenUnconnected=off
  wires:
  AND_Neg/1 -> OR/2
  NOT2/1 -> AND_Neg/2  "negativeDirection"
  OR/1 -> Switch_Stop/2  "stopAccelerating"
  AND_Pos/1 -> OR/1
  NOT1/1 -> AND_Pos/1  "currentGreaterThanTarget"
  Constant/1 -> Switch_Stop/1
  Switch_Dir/1 -> Switch_Stop/3  "accleration"
  Switch_Stop/1 -> accelCommand/1
  Acceleration/1 -> Switch_Dir/1, Unary_Minus/1
  Unary_Minus/1 -> Switch_Dir/3
  Detect Change/1 -> Latch_Target/2
  V_Target/1 -> GreaterThan/1, Detect Change/1
  V_Current/1 -> GreaterThan/2
  GreaterThan/1 -> AND_Neg/1, Latch_Target/1, NOT1/1  "currentLessThanTarget"
  Latch_Target/1 -> NOT2/1, AND_Pos/2, Switch_Dir/2, Unit Delay/1  "positiveDirection"
  Unit Delay/1 -> Latch_Target/3

== system focVelocityEncoder/Controller_Modes/Over_Current_Detector/Subsystem/For Iterator Subsystem ==
  current : Inport
  reset : Inport  Port=2
  Constant : Constant  Value=inverterCurrentMax  OutDataTypeStr=Inherit: Inherit via back propagation
  For Iterator : ForIterator  IterationSource=external  IterationVariableDataType=uint16
  Index Vector : MultiPortSwitch  Inputs=1
  Protection Relay : mcbcontrolslib/Protection Relay  Protection=Overcurrent
      settings: SourceProductBaseCode=MT
  Width : Width  DataType=uint16
  error : Outport  InitialOutput=0
  wires:
  For Iterator/1 -> Index Vector/1
  Index Vector/1 -> Protection Relay/2
  Protection Relay/1 -> error/1
  current/1 -> Width/1, Index Vector/2
  Width/1 -> For Iterator/1
  reset/1 -> Protection Relay/3
  Constant/1 -> Protection Relay/1

== stateflow chart focVelocityEncoder/Controller_Modes/Mode_Scheduler ==
  settings: updateMethod=DISCRETE
  note: Mode Scheduler
  state Enable_Inverter
    state Open_Loop
      state Open_Loop_Command
      state Find_Encoder_Index
    state Calibrate_Encoder_Offset
    state Closed_Loop
    state Disabled
    (default) -> (junction 378)
    (junction 378) -> Open_Loop_Command [order 1] : [commandType == ...
        |  commandTypeEnum.OpenLoop]
    Open_Loop_Command -> Enable_Inverter : [commandType ~= ...
        |  commandTypeEnum.OpenLoop]
    (junction 378) -> (junction 619) [order 2]
    (junction 619) -> (junction 638) [order 1] : [(commandType == ...
        |   commandTypeEnum.CalibrateEncoder) ...
        |  || (calibrateAtStartup ...
        |      && ~encoderOffsetFound) ]
    (junction 638) -> Find_Encoder_Index [order 1] : [~encoderIndexFound]
    (junction 638) -> Calibrate_Encoder_Offset [order 2]
    (junction 619) -> (junction 604) [order 2]
    Find_Encoder_Index -> Calibrate_Encoder_Offset : [encoderIndexFound]
    Calibrate_Encoder_Offset -> Enable_Inverter [order 2] : [commandType ~= ...
        |   commandTypeEnum.CalibrateEncoder]
    Calibrate_Encoder_Offset -> (junction 604) [order 1] : [encoderOffsetFound && ...
        | commandType ~= commandTypeEnum.CalibrateEncoder]
    (junction 604) -> (junction 232)
    (junction 232) -> Closed_Loop [order 1] : [commandType == ...
        |  commandTypeEnum.ClosedLoop]
    Closed_Loop -> Enable_Inverter : [commandType ~= ...
        |  commandTypeEnum.ClosedLoop]
    (junction 232) -> Disabled [order 2]
  state Stand_By
  state Error
  (default) -> Stand_By
  Stand_By -> Enable_Inverter : [motorOn]
  Enable_Inverter -> Stand_By [order 1] : [~motorOn]
  Error -> Stand_By : [~motorOn]
  Enable_Inverter -> Error [order 3] : [commandType ==...
      |  commandTypeEnum.Error]
  Enable_Inverter -> Error [order 2] : [error]
  data: mode output Enum: modeSchedulerEnum; enableInverter output boolean; motorOn input; commandType input; encoderIndexFound input; openLoop output boolean; Find_Encoder_Index output boolean; calibrateEncoder output boolean; closedLoop output boolean; encoderOffsetFound input; error input; calibrateAtStartup local =paramCalibrateAtStartup
